simulink model "Tragenerator"  (R2021a)
settings: Solver=VariableStepAuto  StartTime=0.0  StopTime=100  MaxStep=0.01  RelTol=1e-3
settings Model: Creator=Sirius  LastModifiedBy=Sirius

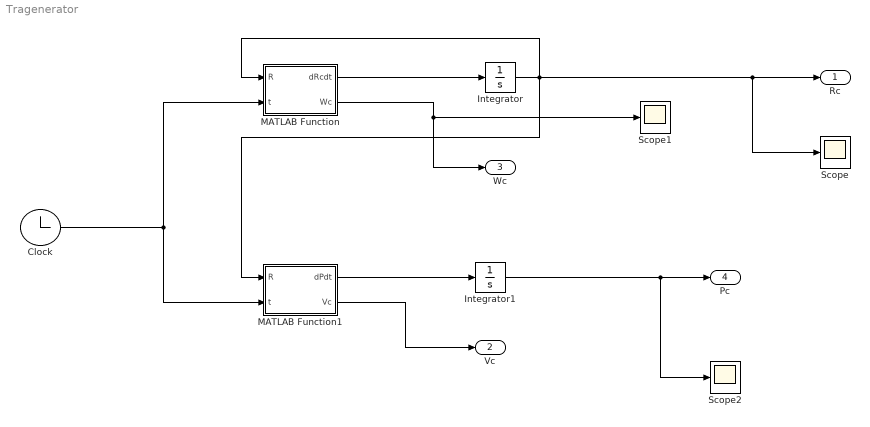
== system Tragenerator ==
  Clock : Clock
  Integrator : Integrator
  Integrator1 : Integrator
  MATLAB Function : MATLAB Function  TreatAsAtomicUnit=on
  MATLAB Function1 : MATLAB Function  TreatAsAtomicUnit=on
  Scope : Scope
  Scope1 : Scope
  Scope2 : Scope
  Rc : Outport
  Vc : Outport  Port=2
  Wc : Outport  Port=3
  Pc : Outport  Port=4
  wires:
  Clock/1 -> MATLAB Function1/2(t), MATLAB Function/2(t)
  MATLAB Function/1(dRcdt) -> Integrator/1
  MATLAB Function/2(Wc) -> Scope1/1, Wc/1
  Integrator/1 -> MATLAB Function1/1(R), MATLAB Function/1(R), Scope/1, Rc/1
  MATLAB Function1/1(dPdt) -> Integrator1/1
  Integrator1/1 -> Scope2/1, Pc/1
  MATLAB Function1/2(Vc) -> Vc/1

== matlab function Tragenerator/MATLAB Function ==
  data: R input; dRcdt output; t input; Wc output
function [dRcdt,Wc] =dRcdt(R,t)

Wc=[0;0;0];
if((t>=19.5)&&(t<=20.5))
    Wc=[0;0;pi/2];
end
if((t>=39.5)&&(t<=40.5))
    Wc=[0;0;pi/2];
end
if((t>=59.5)&&(t<=60.5))
    Wc=[0;0;pi/2];
end
dRcdt=R*Skew(Wc)
end

== matlab function Tragenerator/MATLAB Function1 ==
  data: R input; dPdt output; t input; Vc output
function [dPdt,Vc] = dPdt(R,t)
Vc=[0.5;0;0];
dPdt=R*Vc;
end
